simulink model "FLS"  (R2025a)
settings: Solver=VariableStepAuto  StartTime=0.0  StopTime=10.0  RelTol=1e-3
libraries: fuzblock x1
settings Model: Creator=IMMANDI SRI LIKHITA  LastModifiedBy=IMMANDI SRI LIKHITA

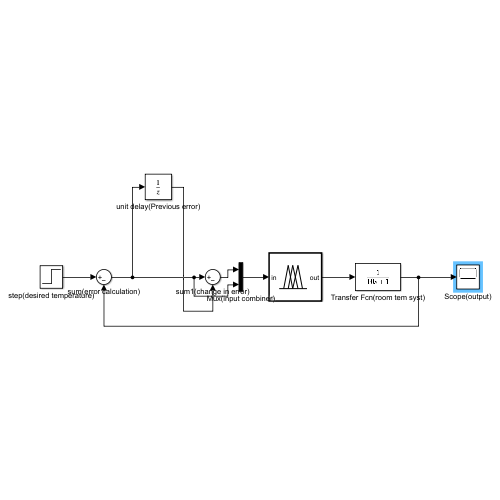
[thumbnail: Simulink's stored preview of the top-level diagram]
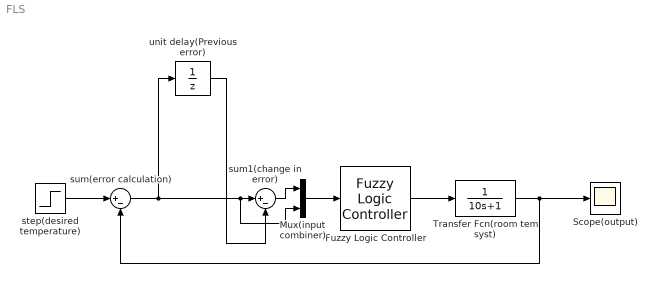
== system FLS ==
  Fuzzy Logic Controller : fuzblock/Fuzzy Logic  Controller  FIS=smart_ac  OutputSampleNumber=101  DataType=double  UseLookupTable=off  NumBreakpoints=10  FuzzifiedInputs=off  RuleFiringStrengths=off  RuleOutputs=off  AggregatedOutputs=off  SimulateUsing=Interpreted execution  OutOfRangeInputValueMessage=warning  NoRuleFiredMessage=warning  EmptyOutputFuzzySetMessage=warning
  Mux(input combiner) : Mux  Inputs=2
  Scope(output) : Scope
      settings: ActiveDisplayYMinimum=-3.6795468164761642  ActiveDisplayYMaximum=33.115921348285482
  Transfer Fcn(room tem syst) : TransferFcn  Denominator=[10 1]
  step(desired temperature) : Step  Time=0  After=5  SampleTime=0
  sum(error calculation) : Sum  Inputs=|+-
  sum1(change in error) : Sum  Inputs=|+-
  unit delay(Previous error) : UnitDelay  SampleTime=-1  StateName=previous error  HasFrameUpgradeWarning=on
  wires:
  step(desired temperature)/1 -> sum(error calculation)/1
  Transfer Fcn(room tem syst)/1 -> sum(error calculation)/2, Scope(output)/1
  Fuzzy Logic Controller/1 -> Transfer Fcn(room tem syst)/1
  sum1(change in error)/1 -> Mux(input combiner)/1
  Mux(input combiner)/1 -> Fuzzy Logic Controller/1
  sum(error calculation)/1 -> unit delay(Previous error)/1, Mux(input combiner)/2, sum1(change in error)/1
  unit delay(Previous error)/1 -> sum1(change in error)/2
